simulink model "nn_fuel_control_6_10"  (R2021a)
settings: Solver=ode15s  StartTime=0.0  StopTime=T  MaxStep=.01  RelTol=1e-3
undefined symbols (not defined in the file): AF_sensor_tol, fault_time, fuel_inj_tol, kappa_tol, MAF_sensor_tol, pump_tol, tau_ww_tol
libraries: neural x68
(part 3 of 3)

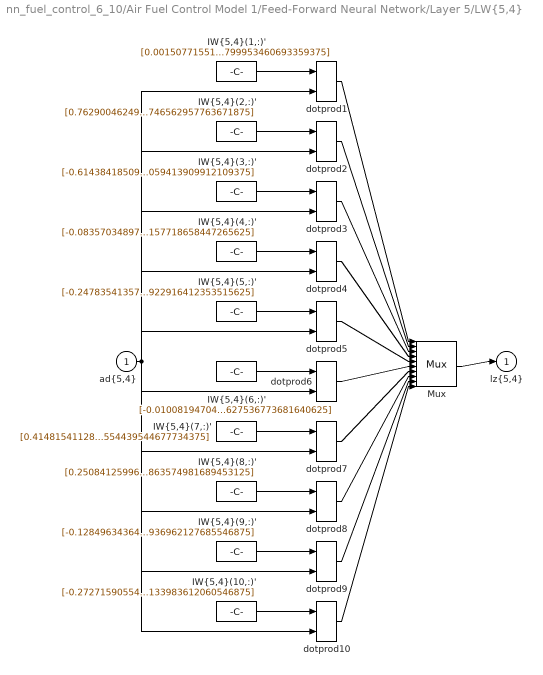
== system nn_fuel_control_6_10/Air Fuel Control Model 1/Feed-Forward Neural Network/Layer 5/LW{5,4} ==
  "ad{5,4}" : Inport  PortDimensions=10
      mask Display: e = 0.06;c1 = [120 230 180]/255;c2 = ([120 230 180]+0)/(256+128);c3 = ([120 230 180]+128)/(256+128);patch([0 1 1 0],[0 0 1 1],c1);patch([0 1 1 1-e 1-e 0+e],[0 0 1 1-e 0+e 0+e],c2);patch([0 0 1 1-e 0+e 0+e],[0 1 1 1-e 1-e 0+e],c3);plot([0 1 1 0 0],[0 0 1 1 0]);
  "IW{5,4}(1,:)'" : Constant  Value=[0.00150771551277439062356544585696838112198747694492340087890625;0.404083630927038972568965391474193893373012542724609375;0.72193388184109685834499714474077336490154266357421875;0.1291915183625412522072650745030841790139675140380859375;-0.5388640868366587621807184405042789876461029052734375;-1.1169862972383561849909483498777262866497039794921875;0.708783347412976549861696184962056577205657958984375;-0.184811990616041921242640455602668225765228271484375;0.47534372063223273574550375997205264866352081298828125;0.360853537334699436822660345569602213799953460693359375]
      mask Display: e = 0.06;c1 = [120 150 230]/255;c2 = ([120 150 230]+0)/383;c3 = ([120 150 230]+128)/383;patch([0 1 1 0],[0 0 1 1],c1);patch([0 1 1 1-e 1-e 0+e],[0 0 1 1-e 0+e 0+e],c2);patch([0 0 1 1-e 0+e 0+e],[0 1 1 1-e 1-e 0+e],c3);plot([0 1 1 0 0],[0 0 1 1 0]);disp('weights');
  "IW{5,4}(10,:)'" : Constant  Value=[-0.272715905544549330752346349981962703168392181396484375;0.693371659950674068539910877007059752941131591796875;0.26697944390492567290351644260226748883724212646484375;-0.224321470291462266022364246964571066200733184814453125;0.472400929639854805230925194337032735347747802734375;1.4695064793347583087523844369570724666118621826171875;0.47273560259150804174765880816266871988773345947265625;-0.568290816901046103026828859583474695682525634765625;0.313597933328539746344887362283770926296710968017578125;0.727304391784552972666233472409658133983612060546875]
      mask Display: e = 0.06;c1 = [120 150 230]/255;c2 = ([120 150 230]+0)/383;c3 = ([120 150 230]+128)/383;patch([0 1 1 0],[0 0 1 1],c1);patch([0 1 1 1-e 1-e 0+e],[0 0 1 1-e 0+e 0+e],c2);patch([0 0 1 1-e 0+e 0+e],[0 1 1 1-e 1-e 0+e],c3);plot([0 1 1 0 0],[0 0 1 1 0]);disp('weights');
  "IW{5,4}(2,:)'" : Constant  Value=[0.762900462490406550131183394114486873149871826171875;0.991309068679945060154068414703942835330963134765625;0.433931623002731636784545798946055583655834197998046875;0.5453508270015190451118769487948156893253326416015625;0.914737780540226363967803990817628800868988037109375;-0.7832881820817652052113544414169155061244964599609375;1.044115230617368439425263204611837863922119140625;0.45468185820289619414324988611042499542236328125;-0.208717972752500369182371287024579942226409912109375;0.010780525598961747391069110335592995397746562957763671875]
      mask Display: e = 0.06;c1 = [120 150 230]/255;c2 = ([120 150 230]+0)/383;c3 = ([120 150 230]+128)/383;patch([0 1 1 0],[0 0 1 1],c1);patch([0 1 1 1-e 1-e 0+e],[0 0 1 1-e 0+e 0+e],c2);patch([0 0 1 1-e 0+e 0+e],[0 1 1 1-e 1-e 0+e],c3);plot([0 1 1 0 0],[0 0 1 1 0]);disp('weights');
  "IW{5,4}(3,:)'" : Constant  Value=[-0.614384185096512158708037532051093876361846923828125;-0.018855747465520600325561417776043526828289031982421875;-0.9912603525906060752959092496894299983978271484375;-0.4070718935054526976813349392614327371120452880859375;0.377276742859228131354853985612862743437290191650390625;0.801605315326323175639799956115894019603729248046875;-0.4193915537095576073767233538092114031314849853515625;0.6165771958938648378278912787209264934062957763671875;-0.121557120783098049354720160408760420978069305419921875;-0.455675653168715333318772309212363325059413909912109375]
      mask Display: e = 0.06;c1 = [120 150 230]/255;c2 = ([120 150 230]+0)/383;c3 = ([120 150 230]+128)/383;patch([0 1 1 0],[0 0 1 1],c1);patch([0 1 1 1-e 1-e 0+e],[0 0 1 1-e 0+e 0+e],c2);patch([0 0 1 1-e 0+e 0+e],[0 1 1 1-e 1-e 0+e],c3);plot([0 1 1 0 0],[0 0 1 1 0]);disp('weights');
  "IW{5,4}(4,:)'" : Constant  Value=[-0.08357034897444137744315639793057925999164581298828125;-0.6579858025992135761583767816773615777492523193359375;-0.13316218445857541663457368485978804528713226318359375;0.34324979081087836352281783547368831932544708251953125;0.3395648969491222857186585315503180027008056640625;-1.0732063928279764741802182470564730465412139892578125;0.399832579454372005756113139796070754528045654296875;0.0584316335549879273258966350113041698932647705078125;-0.8867205172052365913515359352459199726581573486328125;-0.8179601125283488816108956598327495157718658447265625]
      mask Display: e = 0.06;c1 = [120 150 230]/255;c2 = ([120 150 230]+0)/383;c3 = ([120 150 230]+128)/383;patch([0 1 1 0],[0 0 1 1],c1);patch([0 1 1 1-e 1-e 0+e],[0 0 1 1-e 0+e 0+e],c2);patch([0 0 1 1-e 0+e 0+e],[0 1 1 1-e 1-e 0+e],c3);plot([0 1 1 0 0],[0 0 1 1 0]);disp('weights');
  "IW{5,4}(5,:)'" : Constant  Value=[-0.2478354135738121410970080660263192839920520782470703125;-1.0092593029926606451596171609708108007907867431640625;0.06787055085422812050754970414345734752714633941650390625;-0.463032953693297055774991122234496288001537322998046875;0.263659211622163491828274572981172241270542144775390625;-0.79300490423232827819077783715329132974147796630859375;-0.466123491694577507526986437369487248361110687255859375;-0.892927440065978128558299431460909545421600341796875;-0.276041216566703717649744476148043759167194366455078125;-0.191351448543303048754893325167358852922916412353515625]
      mask Display: e = 0.06;c1 = [120 150 230]/255;c2 = ([120 150 230]+0)/383;c3 = ([120 150 230]+128)/383;patch([0 1 1 0],[0 0 1 1],c1);patch([0 1 1 1-e 1-e 0+e],[0 0 1 1-e 0+e 0+e],c2);patch([0 0 1 1-e 0+e 0+e],[0 1 1 1-e 1-e 0+e],c3);plot([0 1 1 0 0],[0 0 1 1 0]);disp('weights');
  "IW{5,4}(6,:)'" : Constant  Value=[-0.01008194704814505647527678178221322013996541500091552734375;-0.09905752911871627819362373656986164860427379608154296875;0.570432190835045371812839221092872321605682373046875;0.305801933958862459661531829624436795711517333984375;-0.2678930180588796616802937933243811130523681640625;1.240487025118707009596619172953069210052490234375;-0.24672430789260368921844701617374084889888763427734375;-0.597026032508149118172013913863338530063629150390625;-0.65440867634247379402978594953310675919055938720703125;-0.2226779515030715972390140677816816605627536773681640625]
      mask Display: e = 0.06;c1 = [120 150 230]/255;c2 = ([120 150 230]+0)/383;c3 = ([120 150 230]+128)/383;patch([0 1 1 0],[0 0 1 1],c1);patch([0 1 1 1-e 1-e 0+e],[0 0 1 1-e 0+e 0+e],c2);patch([0 0 1 1-e 0+e 0+e],[0 1 1 1-e 1-e 0+e],c3);plot([0 1 1 0 0],[0 0 1 1 0]);disp('weights');
  "IW{5,4}(7,:)'" : Constant  Value=[0.414815411282862978037400125685962848365306854248046875;0.43466799027157188017866928930743597447872161865234375;-0.61241216622386585033410710821044631302356719970703125;-0.51301962748979856865361171003314666450023651123046875;-0.482537355779562415758476845439872704446315765380859375;-0.51131234071614095615387896032189019024372100830078125;0.293672962809141846474147996559622697532176971435546875;0.8268111586961068848466993586043827235698699951171875;-1.22053415338308557380742058739997446537017822265625;-1.0191236700273458293253270312561653554439544677734375]
      mask Display: e = 0.06;c1 = [120 150 230]/255;c2 = ([120 150 230]+0)/383;c3 = ([120 150 230]+128)/383;patch([0 1 1 0],[0 0 1 1],c1);patch([0 1 1 1-e 1-e 0+e],[0 0 1 1-e 0+e 0+e],c2);patch([0 0 1 1-e 0+e 0+e],[0 1 1 1-e 1-e 0+e],c3);plot([0 1 1 0 0],[0 0 1 1 0]);disp('weights');
  "IW{5,4}(8,:)'" : Constant  Value=[0.250841259966958773919287750686635263264179229736328125;0.29262474081205935849681054605753161013126373291015625;0.032298514178116848050148490756328101269900798797607421875;-0.466850088900441828609899630464497022330760955810546875;-0.267259419467295644690096878548501990735530853271484375;0.76688348384998039630744415262597613036632537841796875;-1.3483789906671022063022746806382201611995697021484375;-0.2820408410557602163493129410198889672756195068359375;-0.421178631080387055884983737996662966907024383544921875;-0.5244266334925005157430177860078401863574981689453125]
      mask Display: e = 0.06;c1 = [120 150 230]/255;c2 = ([120 150 230]+0)/383;c3 = ([120 150 230]+128)/383;patch([0 1 1 0],[0 0 1 1],c1);patch([0 1 1 1-e 1-e 0+e],[0 0 1 1-e 0+e 0+e],c2);patch([0 0 1 1-e 0+e 0+e],[0 1 1 1-e 1-e 0+e],c3);plot([0 1 1 0 0],[0 0 1 1 0]);disp('weights');
  "IW{5,4}(9,:)'" : Constant  Value=[-0.1284963436482209342415217179222963750362396240234375;0.93483041880704809134527977221296168863773345947265625;-0.091289292745573569209938113999669440090656280517578125;0.7762606349665166494133927699294872581958770751953125;-1.119209383243205291336153095471672713756561279296875;1.2298258097319691994897539188968949019908905029296875;-0.433536551758214871998831085875281132757663726806640625;0.1578262500131877299480720466817729175090789794921875;0.4867239681395465478175310636288486421108245849609375;-0.2112355574267150426504002780347946099936962127685546875]
      mask Display: e = 0.06;c1 = [120 150 230]/255;c2 = ([120 150 230]+0)/383;c3 = ([120 150 230]+128)/383;patch([0 1 1 0],[0 0 1 1],c1);patch([0 1 1 1-e 1-e 0+e],[0 0 1 1-e 0+e 0+e],c2);patch([0 0 1 1-e 0+e 0+e],[0 1 1 1-e 1-e 0+e],c3);plot([0 1 1 0 0],[0 0 1 1 0]);disp('weights');
  Mux : Mux  Inputs=10
      mask Display: e = 0.06;c1 = [120 150 230]/255;c2 = ([120 150 230]+0)/383;c3 = ([120 150 230]+128)/383;patch([0 1 1 0],[0 0 1 1],c1);patch([0 1 1 1-e 1-e 0+e],[0 0 1 1-e 0+e 0+e],c2);patch([0 0 1 1-e 0+e 0+e],[0 1 1 1-e 1-e 0+e],c3);plot([0 1 1 0 0],[0 0 1 1 0]);disp('Mux');
  dotprod{1..10} (10 alike) : neural/Weight Functions/dotprod
  "lz{5,4}" : Outport
      mask Display: e = 0.06;c1 = [120 230 180]/255;c2 = ([120 230 180]+0)/(256+128);c3 = ([120 230 180]+128)/(256+128);patch([0 1 1 0],[0 0 1 1],c1);patch([0 1 1 1-e 1-e 0+e],[0 0 1 1-e 0+e 0+e],c2);patch([0 0 1 1-e 0+e 0+e],[0 1 1 1-e 1-e 0+e],c3);plot([0 1 1 0 0],[0 0 1 1 0]);
  wires:
  "IW{5,4}(1,:)'"/1 -> dotprod1/1
  "ad{5,4}"/1 -> dotprod1/2, dotprod2/2, dotprod3/2, dotprod4/2, dotprod5/2, dotprod6/2, dotprod7/2, dotprod8/2, dotprod9/2, dotprod10/2
  dotprod1/1 -> Mux/1
  "IW{5,4}(2,:)'"/1 -> dotprod2/1
  dotprod2/1 -> Mux/2
  "IW{5,4}(3,:)'"/1 -> dotprod3/1
  dotprod3/1 -> Mux/3
  "IW{5,4}(4,:)'"/1 -> dotprod4/1
  dotprod4/1 -> Mux/4
  "IW{5,4}(5,:)'"/1 -> dotprod5/1
  dotprod5/1 -> Mux/5
  "IW{5,4}(6,:)'"/1 -> dotprod6/1
  dotprod6/1 -> Mux/6
  "IW{5,4}(7,:)'"/1 -> dotprod7/1
  dotprod7/1 -> Mux/7
  "IW{5,4}(8,:)'"/1 -> dotprod8/1
  dotprod8/1 -> Mux/8
  "IW{5,4}(9,:)'"/1 -> dotprod9/1
  dotprod9/1 -> Mux/9
  "IW{5,4}(10,:)'"/1 -> dotprod10/1
  dotprod10/1 -> Mux/10
  Mux/1 -> "lz{5,4}"/1

== system nn_fuel_control_6_10/Air Fuel Control Model 1/Feed-Forward Neural Network/Layer 6/Delays 1 ==
  "p{6}" : Inport  PortDimensions=10
      mask Display: e = 0.06;c1 = [120 230 180]/255;c2 = ([120 230 180]+0)/(256+128);c3 = ([120 230 180]+128)/(256+128);patch([0 1 1 0],[0 0 1 1],c1);patch([0 1 1 1-e 1-e 0+e],[0 0 1 1-e 0+e 0+e],c2);patch([0 0 1 1-e 0+e 0+e],[0 1 1 1-e 1-e 0+e],c3);plot([0 1 1 0 0],[0 0 1 1 0]);
  mux : Mux  Inputs=1
      mask Display: e = 0.06;c1 = [120 150 230]/255;c2 = ([120 150 230]+0)/383;c3 = ([120 150 230]+128)/383;patch([0 1 1 0],[0 0 1 1],c1);patch([0 1 1 1-e 1-e 0+e],[0 0 1 1-e 0+e 0+e],c2);patch([0 0 1 1-e 0+e 0+e],[0 1 1 1-e 1-e 0+e],c3);plot([0 1 1 0 0],[0 0 1 1 0]);disp('Mux')
  "pd{6,5}" : Outport
      mask Display: e = 0.06;c1 = [120 230 180]/255;c2 = ([120 230 180]+0)/(256+128);c3 = ([120 230 180]+128)/(256+128);patch([0 1 1 0],[0 0 1 1],c1);patch([0 1 1 1-e 1-e 0+e],[0 0 1 1-e 0+e 0+e],c2);patch([0 0 1 1-e 0+e 0+e],[0 1 1 1-e 1-e 0+e],c3);plot([0 1 1 0 0],[0 0 1 1 0]);
  wires:
  "p{6}"/1 -> mux/1
  mux/1 -> "pd{6,5}"/1

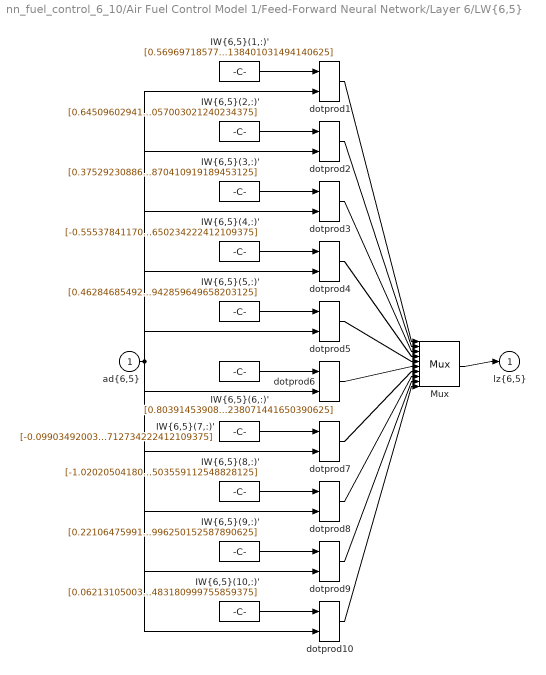
== system nn_fuel_control_6_10/Air Fuel Control Model 1/Feed-Forward Neural Network/Layer 6/LW{6,5} ==
  "ad{6,5}" : Inport  PortDimensions=10
      mask Display: e = 0.06;c1 = [120 230 180]/255;c2 = ([120 230 180]+0)/(256+128);c3 = ([120 230 180]+128)/(256+128);patch([0 1 1 0],[0 0 1 1],c1);patch([0 1 1 1-e 1-e 0+e],[0 0 1 1-e 0+e 0+e],c2);patch([0 0 1 1-e 0+e 0+e],[0 1 1 1-e 1-e 0+e],c3);plot([0 1 1 0 0],[0 0 1 1 0]);
  "IW{6,5}(1,:)'" : Constant  Value=[0.56969718577019368144220834437874145805835723876953125;-0.0225509130740831655048683757058824994601309299468994140625;-0.4834518136891416961731238188804127275943756103515625;1.04416279125057798182751866988837718963623046875;-0.32290613781430799189564595508272759616374969482421875;0.11056254064109817536465385501287528313696384429931640625;-0.82061490378070367501806003929232247173786163330078125;-1.1253378056471798895898928094538860023021697998046875;-0.8886553084147175152196496128453873097896575927734375;0.01261349939040024882574986264671679236926138401031494140625]
      mask Display: e = 0.06;c1 = [120 150 230]/255;c2 = ([120 150 230]+0)/383;c3 = ([120 150 230]+128)/383;patch([0 1 1 0],[0 0 1 1],c1);patch([0 1 1 1-e 1-e 0+e],[0 0 1 1-e 0+e 0+e],c2);patch([0 0 1 1-e 0+e 0+e],[0 1 1 1-e 1-e 0+e],c3);plot([0 1 1 0 0],[0 0 1 1 0]);disp('weights');
  "IW{6,5}(10,:)'" : Constant  Value=[0.062131050031782257547785519591343472711741924285888671875;0.6773248570703984672292108371038921177387237548828125;-0.146135279441022836177666022194898687303066253662109375;-0.603368922165288257275506111909635365009307861328125;0.1738778970152263514403756516912835650146007537841796875;1.04873193011577203748174724751152098178863525390625;-0.03108865148111039644618358579464256763458251953125;-1.2950080224846873822031056988635100424289703369140625;0.4898659650253323061264154603122733533382415771484375;-0.5623207442605104855459785540006123483180999755859375]
      mask Display: e = 0.06;c1 = [120 150 230]/255;c2 = ([120 150 230]+0)/383;c3 = ([120 150 230]+128)/383;patch([0 1 1 0],[0 0 1 1],c1);patch([0 1 1 1-e 1-e 0+e],[0 0 1 1-e 0+e 0+e],c2);patch([0 0 1 1-e 0+e 0+e],[0 1 1 1-e 1-e 0+e],c3);plot([0 1 1 0 0],[0 0 1 1 0]);disp('weights');
  "IW{6,5}(2,:)'" : Constant  Value=[0.6450960294137491057853139864164404571056365966796875;0.68010773815466418756869870776426978409290313720703125;-0.6121139852019894522783260981668718159198760986328125;0.54049636947563584055131968852947466075420379638671875;0.78717152307888493822929376619867980480194091796875;1.053885622547140687998989960760809481143951416015625;0.1483178717150023528947855311344028450548648834228515625;-0.027268084406261335062016115671212901361286640167236328125;0.4121731682278164665689246248803101480007171630859375;-0.72596172762173816206399123984738253057003021240234375]
      mask Display: e = 0.06;c1 = [120 150 230]/255;c2 = ([120 150 230]+0)/383;c3 = ([120 150 230]+128)/383;patch([0 1 1 0],[0 0 1 1],c1);patch([0 1 1 1-e 1-e 0+e],[0 0 1 1-e 0+e 0+e],c2);patch([0 0 1 1-e 0+e 0+e],[0 1 1 1-e 1-e 0+e],c3);plot([0 1 1 0 0],[0 0 1 1 0]);disp('weights');
  "IW{6,5}(3,:)'" : Constant  Value=[0.3752923088679154250968394990195520222187042236328125;-0.71762046978154092613522152532823383808135986328125;-0.6673493066154894126640328977373428642749786376953125;0.973186063116783461879322203458286821842193603515625;0.1242592335000460845861880443408153951168060302734375;-0.90131776509934891095099374069832265377044677734375;-0.006098315875034732158610495389439165592193603515625;0.0829062321821527614673641437548212707042694091796875;0.18759934097352992665719284559600055217742919921875;-0.866493852670505493307473443564958870410919189453125]
      mask Display: e = 0.06;c1 = [120 150 230]/255;c2 = ([120 150 230]+0)/383;c3 = ([120 150 230]+128)/383;patch([0 1 1 0],[0 0 1 1],c1);patch([0 1 1 1-e 1-e 0+e],[0 0 1 1-e 0+e 0+e],c2);patch([0 0 1 1-e 0+e 0+e],[0 1 1 1-e 1-e 0+e],c3);plot([0 1 1 0 0],[0 0 1 1 0]);disp('weights');
  "IW{6,5}(4,:)'" : Constant  Value=[-0.555378411708844499372617065091617405414581298828125;-0.42384351463819414096434456951101310551166534423828125;0.483786539697366235746045504129142500460147857666015625;-0.362552188732002733662085347532411105930805206298828125;1.08828529112606720019584827241487801074981689453125;0.728682458504515739861062684212811291217803955078125;0.5014988797617145888096956696244888007640838623046875;-0.97338054321169564797600060046534053981304168701171875;-3.728031890051120900153591719572432339191436767578125;0.25812211791098282898104798732674680650234222412109375]
      mask Display: e = 0.06;c1 = [120 150 230]/255;c2 = ([120 150 230]+0)/383;c3 = ([120 150 230]+128)/383;patch([0 1 1 0],[0 0 1 1],c1);patch([0 1 1 1-e 1-e 0+e],[0 0 1 1-e 0+e 0+e],c2);patch([0 0 1 1-e 0+e 0+e],[0 1 1 1-e 1-e 0+e],c3);plot([0 1 1 0 0],[0 0 1 1 0]);disp('weights');
  "IW{6,5}(5,:)'" : Constant  Value=[0.462846854925483996989754587048082612454891204833984375;-0.0409250225584348592544614575672312639653682708740234375;0.7322574723543582297935472524841316044330596923828125;-0.304431520859830440084436986580840311944484710693359375;-0.167681221318074891168947715414105914533138275146484375;-0.58135785579806553702297833297052420675754547119140625;-0.90804163297492512807451703338301740586757659912109375;0.5792558966441234691302497594733722507953643798828125;-0.94958564171102022299919553915970027446746826171875;-1.1164234371044312599252634754520840942859649658203125]
      mask Display: e = 0.06;c1 = [120 150 230]/255;c2 = ([120 150 230]+0)/383;c3 = ([120 150 230]+128)/383;patch([0 1 1 0],[0 0 1 1],c1);patch([0 1 1 1-e 1-e 0+e],[0 0 1 1-e 0+e 0+e],c2);patch([0 0 1 1-e 0+e 0+e],[0 1 1 1-e 1-e 0+e],c3);plot([0 1 1 0 0],[0 0 1 1 0]);disp('weights');
  "IW{6,5}(6,:)'" : Constant  Value=[0.80391453908834009656203534177620895206928253173828125;-0.6173290163487621384774683974683284759521484375;-0.561042642012130610140729913837276399135589599609375;-0.4390569380801083720911037744372151792049407958984375;-0.82327700169511863759197467516059987246990203857421875;0.6135960723024964647009937834809534251689910888671875;0.411764143522542980235812137834727764129638671875;0.58198665830650953001423886234988458454608917236328125;-0.294051768416348002777027659249142743647098541259765625;0.385022853218278948705943776076310314238071441650390625]
      mask Display: e = 0.06;c1 = [120 150 230]/255;c2 = ([120 150 230]+0)/383;c3 = ([120 150 230]+128)/383;patch([0 1 1 0],[0 0 1 1],c1);patch([0 1 1 1-e 1-e 0+e],[0 0 1 1-e 0+e 0+e],c2);patch([0 0 1 1-e 0+e 0+e],[0 1 1 1-e 1-e 0+e],c3);plot([0 1 1 0 0],[0 0 1 1 0]);disp('weights');
  "IW{6,5}(7,:)'" : Constant  Value=[-0.0990349200303919097176930108616943471133708953857421875;-0.236441419787699003141057119137258268892765045166015625;0.351954230947536805818032235038117505609989166259765625;0.94378109239855800804974705897620879113674163818359375;4.7335610780795942531540276831947267055511474609375;-1.2749991756659804220674914176925085484981536865234375;0.73692863563723254305415366616216488182544708251953125;3.299601922245816165712994916248135268688201904296875;0.392637760863554119428187050289125181734561920166015625;1.1045060276891793815678965984261594712734222412109375]
      mask Display: e = 0.06;c1 = [120 150 230]/255;c2 = ([120 150 230]+0)/383;c3 = ([120 150 230]+128)/383;patch([0 1 1 0],[0 0 1 1],c1);patch([0 1 1 1-e 1-e 0+e],[0 0 1 1-e 0+e 0+e],c2);patch([0 0 1 1-e 0+e 0+e],[0 1 1 1-e 1-e 0+e],c3);plot([0 1 1 0 0],[0 0 1 1 0]);disp('weights');
  "IW{6,5}(8,:)'" : Constant  Value=[-1.020205041809499224569890429847873747348785400390625;0.317446395325372832108001830420107580721378326416015625;0.7031674645362058218012180077494122087955474853515625;0.603814193628945172775956962141208350658416748046875;1.176203779592970732892354135401546955108642578125;0.25424162268896444150101388004259206354618072509765625;0.29293961175440064170771847784635610878467559814453125;-0.6963573888912175657850411880644969642162322998046875;0.1440748474563888492649965655800770036876201629638671875;-1.1435443692994298192644464506884105503559112548828125]
      mask Display: e = 0.06;c1 = [120 150 230]/255;c2 = ([120 150 230]+0)/383;c3 = ([120 150 230]+128)/383;patch([0 1 1 0],[0 0 1 1],c1);patch([0 1 1 1-e 1-e 0+e],[0 0 1 1-e 0+e 0+e],c2);patch([0 0 1 1-e 0+e 0+e],[0 1 1 1-e 1-e 0+e],c3);plot([0 1 1 0 0],[0 0 1 1 0]);disp('weights');
  "IW{6,5}(9,:)'" : Constant  Value=[0.2210647599175158684037256762167089618742465972900390625;-0.024285736151028081142300152350799180567264556884765625;-0.184122472470563014468325491179712116718292236328125;-0.58768310998157702318422934695263393223285675048828125;0.50642293391728154805520034642540849745273590087890625;-0.47953487519346793543917328861425630748271942138671875;-0.83772158020745857154309987890883348882198333740234375;0.5481901273093325865914948735735379159450531005859375;-0.5363926776671037455201940247206948697566986083984375;-0.60559272859349599915645967485033906996250152587890625]
      mask Display: e = 0.06;c1 = [120 150 230]/255;c2 = ([120 150 230]+0)/383;c3 = ([120 150 230]+128)/383;patch([0 1 1 0],[0 0 1 1],c1);patch([0 1 1 1-e 1-e 0+e],[0 0 1 1-e 0+e 0+e],c2);patch([0 0 1 1-e 0+e 0+e],[0 1 1 1-e 1-e 0+e],c3);plot([0 1 1 0 0],[0 0 1 1 0]);disp('weights');
  Mux : Mux  Inputs=10
      mask Display: e = 0.06;c1 = [120 150 230]/255;c2 = ([120 150 230]+0)/383;c3 = ([120 150 230]+128)/383;patch([0 1 1 0],[0 0 1 1],c1);patch([0 1 1 1-e 1-e 0+e],[0 0 1 1-e 0+e 0+e],c2);patch([0 0 1 1-e 0+e 0+e],[0 1 1 1-e 1-e 0+e],c3);plot([0 1 1 0 0],[0 0 1 1 0]);disp('Mux');
  dotprod{1..10} (10 alike) : neural/Weight Functions/dotprod
  "lz{6,5}" : Outport
      mask Display: e = 0.06;c1 = [120 230 180]/255;c2 = ([120 230 180]+0)/(256+128);c3 = ([120 230 180]+128)/(256+128);patch([0 1 1 0],[0 0 1 1],c1);patch([0 1 1 1-e 1-e 0+e],[0 0 1 1-e 0+e 0+e],c2);patch([0 0 1 1-e 0+e 0+e],[0 1 1 1-e 1-e 0+e],c3);plot([0 1 1 0 0],[0 0 1 1 0]);
  wires:
  "IW{6,5}(1,:)'"/1 -> dotprod1/1
  "ad{6,5}"/1 -> dotprod1/2, dotprod2/2, dotprod3/2, dotprod4/2, dotprod5/2, dotprod6/2, dotprod7/2, dotprod8/2, dotprod9/2, dotprod10/2
  dotprod1/1 -> Mux/1
  "IW{6,5}(2,:)'"/1 -> dotprod2/1
  dotprod2/1 -> Mux/2
  "IW{6,5}(3,:)'"/1 -> dotprod3/1
  dotprod3/1 -> Mux/3
  "IW{6,5}(4,:)'"/1 -> dotprod4/1
  dotprod4/1 -> Mux/4
  "IW{6,5}(5,:)'"/1 -> dotprod5/1
  dotprod5/1 -> Mux/5
  "IW{6,5}(6,:)'"/1 -> dotprod6/1
  dotprod6/1 -> Mux/6
  "IW{6,5}(7,:)'"/1 -> dotprod7/1
  dotprod7/1 -> Mux/7
  "IW{6,5}(8,:)'"/1 -> dotprod8/1
  dotprod8/1 -> Mux/8
  "IW{6,5}(9,:)'"/1 -> dotprod9/1
  dotprod9/1 -> Mux/9
  "IW{6,5}(10,:)'"/1 -> dotprod10/1
  dotprod10/1 -> Mux/10
  Mux/1 -> "lz{6,5}"/1

== system nn_fuel_control_6_10/Air Fuel Control Model 1/Feed-Forward Neural Network/Layer 7/Delays 1 ==
  "p{7}" : Inport  PortDimensions=10
      mask Display: e = 0.06;c1 = [120 230 180]/255;c2 = ([120 230 180]+0)/(256+128);c3 = ([120 230 180]+128)/(256+128);patch([0 1 1 0],[0 0 1 1],c1);patch([0 1 1 1-e 1-e 0+e],[0 0 1 1-e 0+e 0+e],c2);patch([0 0 1 1-e 0+e 0+e],[0 1 1 1-e 1-e 0+e],c3);plot([0 1 1 0 0],[0 0 1 1 0]);
  mux : Mux  Inputs=1
      mask Display: e = 0.06;c1 = [120 150 230]/255;c2 = ([120 150 230]+0)/383;c3 = ([120 150 230]+128)/383;patch([0 1 1 0],[0 0 1 1],c1);patch([0 1 1 1-e 1-e 0+e],[0 0 1 1-e 0+e 0+e],c2);patch([0 0 1 1-e 0+e 0+e],[0 1 1 1-e 1-e 0+e],c3);plot([0 1 1 0 0],[0 0 1 1 0]);disp('Mux')
  "pd{7,6}" : Outport
      mask Display: e = 0.06;c1 = [120 230 180]/255;c2 = ([120 230 180]+0)/(256+128);c3 = ([120 230 180]+128)/(256+128);patch([0 1 1 0],[0 0 1 1],c1);patch([0 1 1 1-e 1-e 0+e],[0 0 1 1-e 0+e 0+e],c2);patch([0 0 1 1-e 0+e 0+e],[0 1 1 1-e 1-e 0+e],c3);plot([0 1 1 0 0],[0 0 1 1 0]);
  wires:
  "p{7}"/1 -> mux/1
  mux/1 -> "pd{7,6}"/1

== system nn_fuel_control_6_10/Air Fuel Control Model 1/Feed-Forward Neural Network/Layer 7/LW{7,6} ==
  "ad{7,6}" : Inport  PortDimensions=10
      mask Display: e = 0.06;c1 = [120 230 180]/255;c2 = ([120 230 180]+0)/(256+128);c3 = ([120 230 180]+128)/(256+128);patch([0 1 1 0],[0 0 1 1],c1);patch([0 1 1 1-e 1-e 0+e],[0 0 1 1-e 0+e 0+e],c2);patch([0 0 1 1-e 0+e 0+e],[0 1 1 1-e 1-e 0+e],c3);plot([0 1 1 0 0],[0 0 1 1 0]);
  "IW{7,6}(1,:)'" : Constant  Value=[0.27832800362124399118357587212813086807727813720703125;0.262682532443176075531710012000985443592071533203125;0.3324960408461750116515531772165559232234954833984375;0.453094279998485560678744832330266945064067840576171875;-0.7707620616369172950044230674393475055694580078125;0.497028666485325787416371667859493754804134368896484375;0.0282633443900698021200579290734822279773652553558349609375;-0.43341886966427356497888467856682837009429931640625;-0.419675895166071899478055229337769560515880584716796875;0.1539047196867997235880665130025590769946575164794921875]
      mask Display: e = 0.06;c1 = [120 150 230]/255;c2 = ([120 150 230]+0)/383;c3 = ([120 150 230]+128)/383;patch([0 1 1 0],[0 0 1 1],c1);patch([0 1 1 1-e 1-e 0+e],[0 0 1 1-e 0+e 0+e],c2);patch([0 0 1 1-e 0+e 0+e],[0 1 1 1-e 1-e 0+e],c3);plot([0 1 1 0 0],[0 0 1 1 0]);disp('weights');
  Mux : Mux  Inputs=1
      mask Display: e = 0.06;c1 = [120 150 230]/255;c2 = ([120 150 230]+0)/383;c3 = ([120 150 230]+128)/383;patch([0 1 1 0],[0 0 1 1],c1);patch([0 1 1 1-e 1-e 0+e],[0 0 1 1-e 0+e 0+e],c2);patch([0 0 1 1-e 0+e 0+e],[0 1 1 1-e 1-e 0+e],c3);plot([0 1 1 0 0],[0 0 1 1 0]);disp('Mux');
  dotprod1 : neural/Weight Functions/dotprod
  "lz{7,6}" : Outport
      mask Display: e = 0.06;c1 = [120 230 180]/255;c2 = ([120 230 180]+0)/(256+128);c3 = ([120 230 180]+128)/(256+128);patch([0 1 1 0],[0 0 1 1],c1);patch([0 1 1 1-e 1-e 0+e],[0 0 1 1-e 0+e 0+e],c2);patch([0 0 1 1-e 0+e 0+e],[0 1 1 1-e 1-e 0+e],c3);plot([0 1 1 0 0],[0 0 1 1 0]);
  wires:
  "IW{7,6}(1,:)'"/1 -> dotprod1/1
  "ad{7,6}"/1 -> dotprod1/2
  dotprod1/1 -> Mux/1
  Mux/1 -> "lz{7,6}"/1
